simulink model "CHM2ActiveSubStateCtrl"  (R2018b)
settings: Solver=FixedStepDiscrete  StartTime=0.0  StopTime=10.0  FixedStep=0.01  RelTol=1e-3
undefined symbols (not defined in the file or in its folder): KeSMSuChmReqDurnTm_Val, KeSMSuChmReqIntlTm_Val
settings Model: Creator=sn2xws  LastModifiedBy=sn2xws
settings DataIOCC: SaveFormat=StructureWithTime
settings OptimizationCC: DefaultParameterBehavior=Inlined  EnhancedBackFolding=on  PassReuseOutputArgsAs=Individual arguments  ZeroExternalMemoryAtStartup=off  ZeroInternalMemoryAtStartup=off  OptimizeBlockOrder=speed  DifferentSizesBufferReuse=on  OptimizationCustomize=off
settings DebuggingCC: ParameterTunabilityLossMsg=error
settings ModelReferenceCC: ModelReferenceNumInstancesAllowed=Single
settings SFSimCC: MATLABDynamicMemAlloc=off
settings RTWCC: SystemTargetFile=autosar.tlc  GenCodeOnly=on  TemplateMakefile=ert_default_tmf  Description=AUTOSAR  GenerateReport=on  IncludeHyperlinkInReport=on  LaunchReport=on  GenerateTraceInfo=on  GenerateTraceReport=on  GenerateTraceReportSl=on  GenerateTraceReportSf=on  GenerateTraceReportEml=on  GenerateCodeMetricsReport=on
settings CodeAppCC: ForceParamTrailComments=on  IgnoreCustomStorageClasses=off  OperatorAnnotations=on  SimulinkDataObjDesc=on  SFDataObjDesc=on  InsertBlockDesc=on
settings STFCustomTargetCC: TargetLangStandard=C99 (ISO)  MultiwordLength=256  ParMdlRefBuildCompliant=on  CompOptLevelCompliant=on  IncludeMdlTerminateFcn=off  CombineOutputUpdateFcns=on  SuppressErrorStatus=on  ERTCustomFileBanners=on  SupportNonFinite=off  SupportComplex=off  SupportContinuousTime=off  SupportNonInlinedSFcns=off  RemoveResetFunc=on  MATLABClassNameForMDSCustomization=Simulink.SoftwareTarget.ERTCustomization  AutosarCompliant=on  UseToolchainInfoCompliant=on  LookupTableObjectStructAxisOrder=2,1,3,4,...  LUTObjectStructOrderEvenSpacing=Size,Table,Breakpoints  SystemTargetFile=autosar.tlc
settings ERTTargetCC: TargetLangStandard=C99 (ISO)  ConcurrentExecutionCompliant=off  IncludeMdlTerminateFcn=off  SuppressErrorStatus=on  SupportNonFinite=off  SupportComplex=off  ModelStepFunctionPrototypeControlCompliant=off  CPPClassGenCompliant=off  AutosarCompliant=on  LookupTableObjectStructAxisOrder=2,1,3,4,...  LUTObjectStructOrderEvenSpacing=Size,Table,Breakpoints  InlinedParameterPlacement=NonHierarchical  ERTCustomFileTemplate=example_file_process.tlc  ERTFilePackagingFormat=Compact

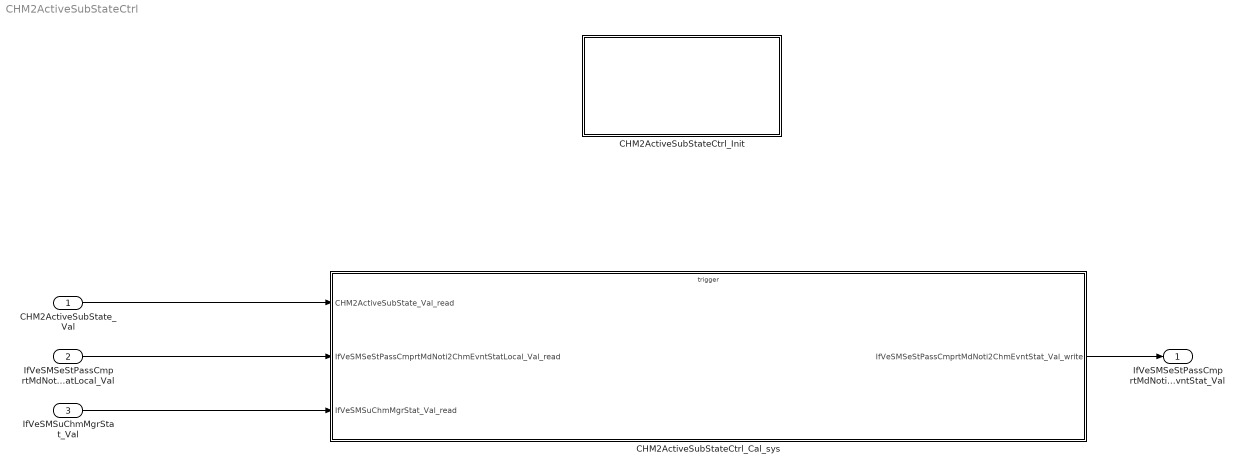
== system CHM2ActiveSubStateCtrl ==
  CHM2ActiveSubState_Val : Inport  OutDataTypeStr=boolean  PortDimensions=1
  IfVeSMSeStPassCmprtMdNoti2ChmEvntStatLocal_Val : Inport  Port=2  OutDataTypeStr=Enum: EventSts1  PortDimensions=1
  IfVeSMSuChmMgrStat_Val : Inport  Port=3  OutDataTypeStr=uint16  PortDimensions=1
  CHM2ActiveSubStateCtrl_Cal_sys : Subsystem
  CHM2ActiveSubStateCtrl_Init : Subsystem
  IfVeSMSeStPassCmprtMdNoti2ChmEvntStat_Val : Outport  OutDataTypeStr=Enum: EventSts1  PortDimensions=1
  wires:
  CHM2ActiveSubState_Val/1 -> CHM2ActiveSubStateCtrl_Cal_sys/1(CHM2ActiveSubState_Val_read)
  IfVeSMSeStPassCmprtMdNoti2ChmEvntStatLocal_Val/1 -> CHM2ActiveSubStateCtrl_Cal_sys/2(IfVeSMSeStPassCmprtMdNoti2ChmEvntStatLocal_Val_read)
  IfVeSMSuChmMgrStat_Val/1 -> CHM2ActiveSubStateCtrl_Cal_sys/3(IfVeSMSuChmMgrStat_Val_read)
  CHM2ActiveSubStateCtrl_Cal_sys/1(IfVeSMSeStPassCmprtMdNoti2ChmEvntStat_Val_write) -> IfVeSMSeStPassCmprtMdNoti2ChmEvntStat_Val/1

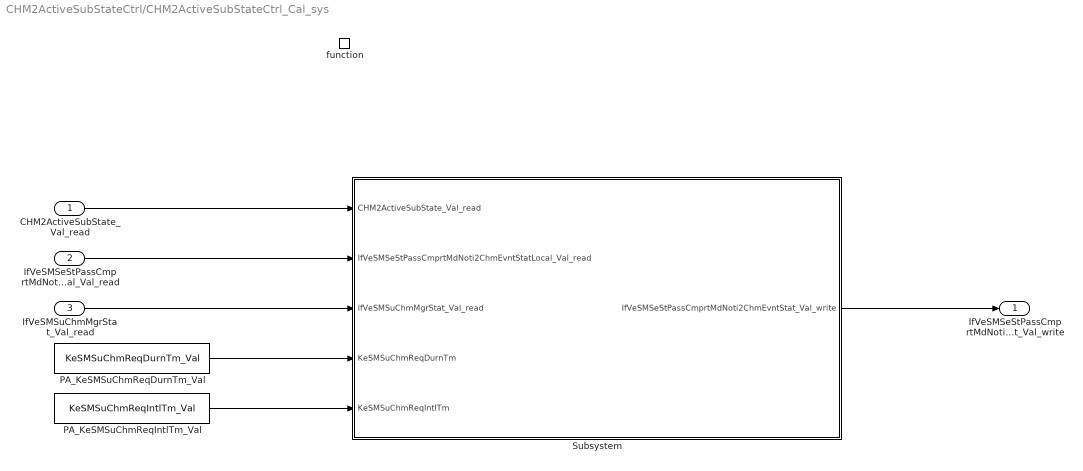
== system CHM2ActiveSubStateCtrl/CHM2ActiveSubStateCtrl_Cal_sys ==
  CHM2ActiveSubState_Val_read : Inport
  IfVeSMSeStPassCmprtMdNoti2ChmEvntStatLocal_Val_read : Inport  Port=2
  IfVeSMSuChmMgrStat_Val_read : Inport  Port=3
  function : TriggerPort  TriggerType=function-call  IsSimulinkFunction=on  FunctionName=CHM2ActiveSubStateCtrl_Cal  VariantControl=(inherit)
  PA_KeSMSuChmReqDurnTm_Val : Constant  Value=KeSMSuChmReqDurnTm_Val
  PA_KeSMSuChmReqIntlTm_Val : Constant  Value=KeSMSuChmReqIntlTm_Val
  Subsystem : Subsystem
  IfVeSMSeStPassCmprtMdNoti2ChmEvntStat_Val_write : Outport
      settings: EnsureOutportIsVirtual=on
  wires:
  CHM2ActiveSubState_Val_read/1 -> Subsystem/1(CHM2ActiveSubState_Val_read)
  PA_KeSMSuChmReqDurnTm_Val/1 -> Subsystem/4(KeSMSuChmReqDurnTm)
  PA_KeSMSuChmReqIntlTm_Val/1 -> Subsystem/5(KeSMSuChmReqIntlTm)
  Subsystem/1(IfVeSMSeStPassCmprtMdNoti2ChmEvntStat_Val_write) -> IfVeSMSeStPassCmprtMdNoti2ChmEvntStat_Val_write/1
  IfVeSMSuChmMgrStat_Val_read/1 -> Subsystem/3(IfVeSMSuChmMgrStat_Val_read)
  IfVeSMSeStPassCmprtMdNoti2ChmEvntStatLocal_Val_read/1 -> Subsystem/2(IfVeSMSeStPassCmprtMdNoti2ChmEvntStatLocal_Val_read)

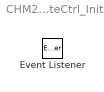
== system CHM2ActiveSubStateCtrl/CHM2ActiveSubStateCtrl_Init ==
  Event Listener : EventListener  EventName=reset

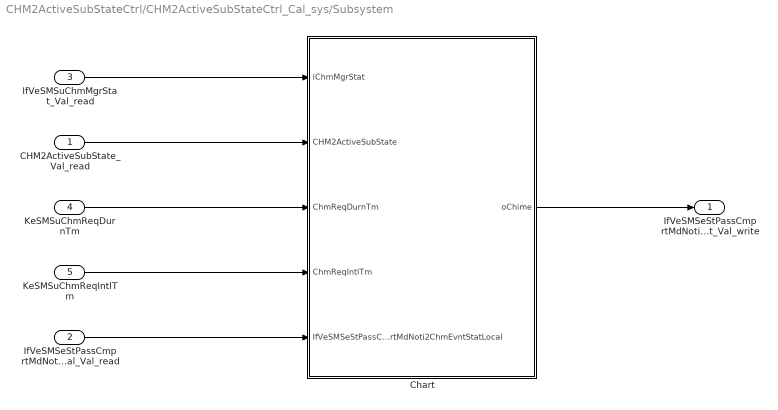
== system CHM2ActiveSubStateCtrl/CHM2ActiveSubStateCtrl_Cal_sys/Subsystem ==
  CHM2ActiveSubState_Val_read : Inport
  IfVeSMSeStPassCmprtMdNoti2ChmEvntStatLocal_Val_read : Inport  Port=2
  IfVeSMSuChmMgrStat_Val_read : Inport  Port=3
  KeSMSuChmReqDurnTm : Inport  Port=4
  KeSMSuChmReqIntlTm : Inport  Port=5
  Chart : Stateflow chart  TreatAsAtomicUnit=on
  IfVeSMSeStPassCmprtMdNoti2ChmEvntStat_Val_write : Outport
      settings: EnsureOutportIsVirtual=on
  wires:
  IfVeSMSuChmMgrStat_Val_read/1 -> Chart/1(iChmMgrStat)
  CHM2ActiveSubState_Val_read/1 -> Chart/2(CHM2ActiveSubState)
  Chart/1(oChime) -> IfVeSMSeStPassCmprtMdNoti2ChmEvntStat_Val_write/1
  KeSMSuChmReqDurnTm/1 -> Chart/3(ChmReqDurnTm)
  KeSMSuChmReqIntlTm/1 -> Chart/4(ChmReqIntlTm)
  IfVeSMSeStPassCmprtMdNoti2ChmEvntStatLocal_Val_read/1 -> Chart/5(IfVeSMSeStPassCmprtMdNoti2ChmEvntStatLocal)

== stateflow chart CHM2ActiveSubStateCtrl/CHM2ActiveSubStateCtrl_Cal_sys/Subsystem/Chart ==
  state CHM2ActiveSubStateOff
    en:oChime = IfVeSMSeStPassCmprtMdNoti2ChmEvntStatLocal;
    du:oChime = IfVeSMSeStPassCmprtMdNoti2ChmEvntStatLocal;
  state CHM2ActiveSubStateOn
    en:retrycnt=0;
    state Idle
      en:
      oChime = EventSts1.EventSts_NoAct;
    state Active1
      en:
      oChime = EventSts1.EventSts_Act;
    (default) -> Idle
    Active1 -> Idle [order 2] : [iChmMgrStat==2725||...
        | iChmMgrStat==0]
    Active1 -> Idle [order 1] : [after(ChmReqDurnTm/10,tick)]
        | {retrycnt=retrycnt+1;}
    Idle -> Active1 : [iChmMgrStat !=0&&iChmMgrStat!=2725&&retrycnt<4&&after(ChmReqIntlTm/10,tick)]
  note: $0=NO_ACTION; $1=ACTIVE; $2=CANCEL_CHIME
  CHM2ActiveSubStateOn -> CHM2ActiveSubStateOn [order 1] : [hasChanged(iChmMgrStat)&&iChmMgrStat!=0&&iChmMgrStat!=2725]
  (default) -> CHM2ActiveSubStateOff
  CHM2ActiveSubStateOff -> CHM2ActiveSubStateOn : [CHM2ActiveSubState]
  CHM2ActiveSubStateOn -> CHM2ActiveSubStateOff [order 2] : [!CHM2ActiveSubState]
  data: iChmMgrStat input; CHM2ActiveSubState input boolean; oChime output Enum: EventSts1; retrycnt local uint8; ChmReqDurnTm input uint8; ChmReqIntlTm input uint8; IfVeSMSeStPassCmprtMdNoti2ChmEvntStatLocal input Enum: EventSts1
